simulink model "CrCUI"  (R2016b)
settings: configuration reference "CodeGenConfigSet" (kept outside this file)
values from neighbouring files (symbols this model uses):
  CrCLmp_nLmpTst_C = Calibration.Parameter    [init_CrCUI.m]
  CRCLMP_NORMAL = fi(80,State_uint8)    [init_CrCUI.m]
  CRCLMP_OFF = fi(40,State_uint8)    [init_CrCUI.m]
  CRCLMP_ON = fi(20,State_uint8)    [init_CrCUI.m]
  CrCLmp_tiLmpTstMax_C = Calibration.Parameter    [init_CrCUI.m]
  CrCLmp_tiLmpTstOff_C = Calibration.Parameter    [init_CrCUI.m]
  CrCLmp_tiLmpTstOn_C = Calibration.Parameter    [init_CrCUI.m]
  CRCLMP_VISUAL = fi(10,State_uint8)    [init_CrCUI.m]
  CrCtl_swtAllwSetDrngOvrd_C = Calibration.Parameter    [init_CrCUI.m]
  CrCUI_tiNeutrPosChk_C = Calibration.Parameter    [init_CrCUI.m]
  CrCUI_tiNeutrStr_C = Calibration.Parameter    [init_CrCUI.m]
  CrCUI_tiSwtActvThres_C = Calibration.Parameter    [init_CrCUI.m]
  CrCUI_tiSwtSetThres_C = Calibration.Parameter    [init_CrCUI.m]
undefined symbols (not defined in the file or in its folder): CrCtl_stOpFunc_conv, CrCtl_stShOff_conv, CrCUI_BttnState_conv, CrCUI_DT, CruiseCtl_State_conv, HLSDem_State_conv, Switch_conv, WESDem_State_conv
libraries: CXLib x17, simulink x14
settings Model: Creator=guanxiaoxing  LastModifiedBy=guanxiaoxing
settings ConfigSetRef: SourceLocation=Base Workspace

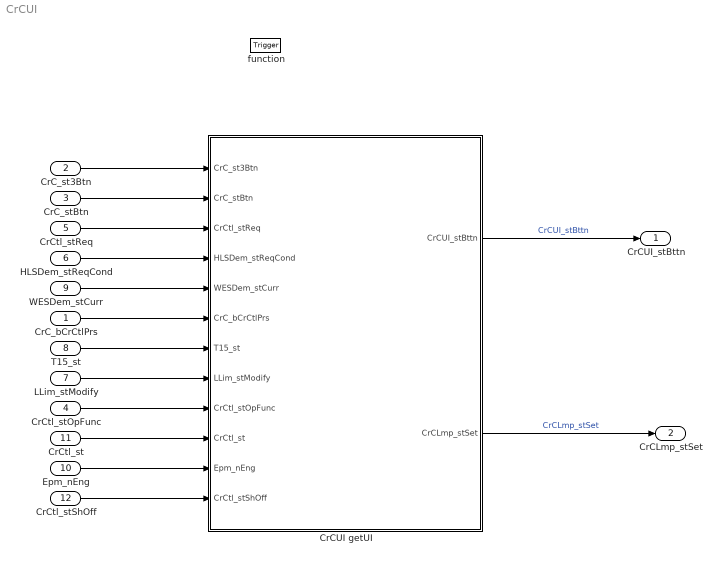
== system CrCUI ==
  CrC_bCrCtlPrs : Inport  Description=Cruise control present status  OutMin=0  OutMax=1  OutDataTypeStr=boolean
  CrC_st3Btn : Inport  Description=two sources for the 3/4 button logic information  Port=2  OutMin=0  OutMax=1  OutDataTypeStr=boolean
  CrC_stBtn : Inport  Description=Status Button Information incase of 3-button logic  Port=3  OutMin=0  OutMax=255  OutDataTypeStr=State_uint8
  CrCtl_stOpFunc : Inport  Description=state of cruise control operation functionality  Port=4  OutDataTypeStr=Enum: CrCtl_stOpFunc_conv
  CrCtl_stReq : Inport  Description=Cruise control is active  Port=5  OutMin=0  OutMax=1  OutDataTypeStr=boolean
  HLSDem_stReqCond : Inport  Description=Status of request for idle speed increase  Port=6  OutMin=0  OutMax=255  OutDataTypeStr=State_uint8
  LLim_stModify : Inport  Description=|  Port=7  OutMin=0  OutMax=1  OutDataTypeStr=boolean
      | Application parameter for Status for changing adjustable
      | vehicle speed limit
  T15_st : Inport  Description=Terminal 15 status after denouncing  Port=8  OutDataTypeStr=Enum: Switch_conv
  WESDem_stCurr : Inport  Description=Status of the working engine Speed Control  Port=9  OutDataTypeStr=Enum: WESDem_State_conv
  Epm_nEng : Inport  Tag=rpm  Description=Engine speed  Port=10  OutMin=0  OutMax=6000  OutDataTypeStr=EngSpeed_rpm
  CrCtl_st : Inport  Description=Application parameter for Cruise Control state  Port=11  OutDataTypeStr=Enum: CruiseCtl_State_conv
  CrCtl_stShOff : Inport  Description=cruise control shut-off requirement  Port=12  OutDataTypeStr=Enum: CrCtl_stShOff_conv
  function : TriggerPort  TriggerType=function-call  VariantControl=Variant
  CrCUI getUI : Subsystem
  CrCUI_stBttn : Outport  Description=Application parameter for status button information  OutDataTypeStr=Enum: CrCUI_BttnState_conv
  CrCLmp_stSet : Outport  Description=input from ASW for cruise set lamp ON/OFF  Port=2  OutMin=0  OutMax=1  OutDataTypeStr=boolean
  wires:
  CrCUI getUI/1(CrCUI_stBttn) -> CrCUI_stBttn/1  "CrCUI_stBttn"
  CrC_st3Btn/1 -> CrCUI getUI/1(CrC_st3Btn)
  CrC_stBtn/1 -> CrCUI getUI/2(CrC_stBtn)
  CrCtl_stReq/1 -> CrCUI getUI/3(CrCtl_stReq)
  HLSDem_stReqCond/1 -> CrCUI getUI/4(HLSDem_stReqCond)
  WESDem_stCurr/1 -> CrCUI getUI/5(WESDem_stCurr)
  T15_st/1 -> CrCUI getUI/7(T15_st)
  CrC_bCrCtlPrs/1 -> CrCUI getUI/6(CrC_bCrCtlPrs)
  CrCtl_stOpFunc/1 -> CrCUI getUI/9(CrCtl_stOpFunc)
  LLim_stModify/1 -> CrCUI getUI/8(LLim_stModify)
  CrCUI getUI/2(CrCLmp_stSet) -> CrCLmp_stSet/1  "CrCLmp_stSet"
  Epm_nEng/1 -> CrCUI getUI/11(Epm_nEng)
  CrCtl_st/1 -> CrCUI getUI/10(CrCtl_st)
  CrCtl_stShOff/1 -> CrCUI getUI/12(CrCtl_stShOff)

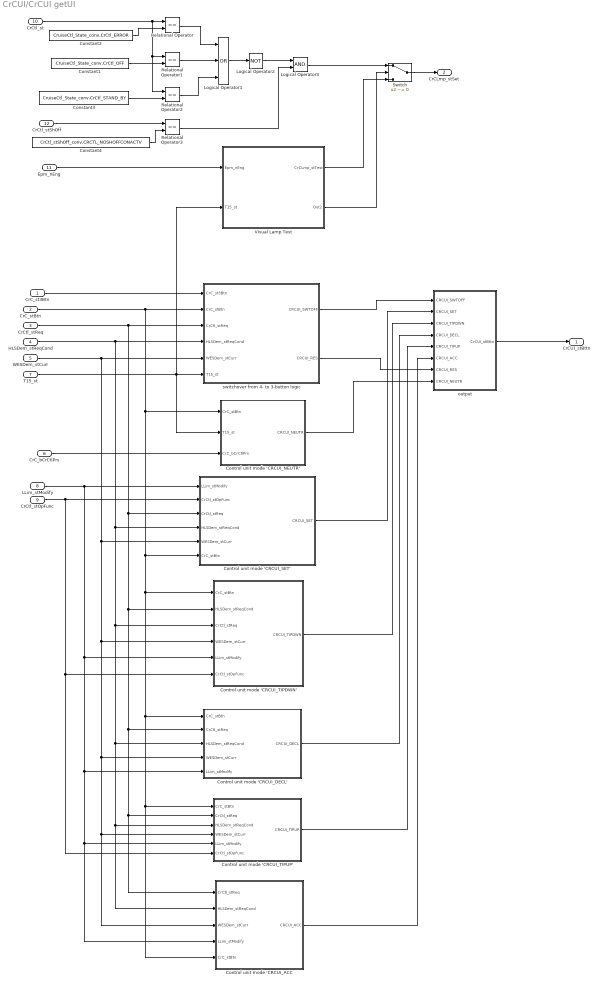
== system CrCUI/CrCUI getUI ==
  CrC_st3Btn : Inport
  CrC_stBtn : Inport  Port=2
  CrCtl_stReq : Inport  Port=3
  HLSDem_stReqCond : Inport  Port=4
  WESDem_stCurr : Inport  Port=5
  CrC_bCrCtlPrs : Inport  Port=6
  T15_st : Inport  Port=7
  LLim_stModify : Inport  Port=8
  CrCtl_stOpFunc : Inport  Port=9
  CrCtl_st : Inport  Port=10
  Epm_nEng : Inport  Port=11
  CrCtl_stShOff : Inport  Port=12
  Constant1 : Constant  Value=CruiseCtl_State_conv.CrCtl_OFF
  Constant2 : Constant  Value=CruiseCtl_State_conv.CrCtl_ERROR
  Constant3 : Constant  Value=CruiseCtl_State_conv.CrCtl_STAND_BY
  Constant4 : Constant  Value=CrCtl_stShOff_conv.CRCTL_NOSHOFFCONACTV
  Control unit mode 'CRCUI_ACC : Subsystem
  Control unit mode 'CRCUI_DECL' : Subsystem
  Control unit mode 'CRCUI_NEUTR' : Subsystem
  Control unit mode 'CRCUI_SET‘ : Subsystem
  Control unit mode 'CRCUI_TIPDWN' : Subsystem
  Control unit mode 'CRCUI_TIPUP' : Subsystem
  Logical Operator1 : Logic  Operator=OR  Inputs=3  AllPortsSameDT=off  OutDataTypeStr=boolean
  Logical Operator2 : Logic  Operator=NOT  AllPortsSameDT=off  OutDataTypeStr=boolean
  Logical Operator3 : Logic  AllPortsSameDT=off  OutDataTypeStr=boolean
  Relational Operator{,1..3} (4 alike) : RelationalOperator  Operator===  OutDataTypeStr=boolean  RndMeth=Simplest
  Switch : Switch  Criteria=u2 ~= 0
  Visual Lamp Test : Subsystem
  output : Subsystem
  switchover from 4- to 3-button logic : Subsystem
  CrCUI_stBttn : Outport
  CrCLmp_stSet : Outport  Port=2
  wires:
  switchover from 4- to 3-button logic/1(CRCUI_SWTOFF) -> output/1(CRCUI_SWTOFF)
  Control unit mode 'CRCUI_SET‘/1(CRCUI_SET) -> output/2(CRCUI_SET)
  Control unit mode 'CRCUI_TIPDWN'/1(CRCUI_TIPDWN) -> output/3(CRCUI_TIPDWN)
  Control unit mode 'CRCUI_DECL'/1(CRCUI_DECL) -> output/4(CRCUI_DECL)
  Control unit mode 'CRCUI_TIPUP'/1(CRCUI_TIPUP) -> output/5(CRCUI_TIPUP)
  Control unit mode 'CRCUI_ACC/1(CRCUI_ACC) -> output/6(CRCUI_ACC)
  switchover from 4- to 3-button logic/2(CRCUI_RES) -> output/7(CRCUI_RES)
  Control unit mode 'CRCUI_NEUTR'/1(CRCUI_NEUTR) -> output/8(CRCUI_NEUTR)
  CrC_st3Btn/1 -> switchover from 4- to 3-button logic/1(CrC_st3Btn)
  CrC_bCrCtlPrs/1 -> Control unit mode 'CRCUI_NEUTR'/3(CrC_bCrCtlPrs)
  CrCtl_stOpFunc/1 -> Control unit mode 'CRCUI_TIPUP'/6(CrCtl_stOpFunc), Control unit mode 'CRCUI_TIPDWN'/6(CrCtl_stOpFunc), Control unit mode 'CRCUI_SET‘/2(CrCtl_stOpFunc)
  LLim_stModify/1 -> Control unit mode 'CRCUI_ACC/4(LLim_stModify), Control unit mode 'CRCUI_TIPUP'/5(LLim_stModify), Control unit mode 'CRCUI_DECL'/5(LLim_stModify), Control unit mode 'CRCUI_TIPDWN'/5(LLim_stModify), Control unit mode 'CRCUI_SET‘/1(LLim_stModify)
  CrCtl_stReq/1 -> Control unit mode 'CRCUI_DECL'/2(CrCtl_stReq), Control unit mode 'CRCUI_TIPUP'/2(CrCtl_stReq), Control unit mode 'CRCUI_ACC/1(CrCtl_stReq), Control unit mode 'CRCUI_TIPDWN'/2(HLSDem_stReqCond), Control unit mode 'CRCUI_SET‘/3(CrCtl_stReq), switchover from 4- to 3-button logic/3(CrCtl_stReq)
  HLSDem_stReqCond/1 -> Control unit mode 'CRCUI_DECL'/3(HLSDem_stReqCond), Control unit mode 'CRCUI_ACC/2(HLSDem_stReqCond), Control unit mode 'CRCUI_TIPUP'/3(HLSDem_stReqCond), Control unit mode 'CRCUI_TIPDWN'/3(CrCtl_stReq), Control unit mode 'CRCUI_SET‘/4(HLSDem_stReqCond), switchover from 4- to 3-button logic/4(HLSDem_stReqCond)
  WESDem_stCurr/1 -> Control unit mode 'CRCUI_ACC/3(WESDem_stCurr), Control unit mode 'CRCUI_TIPUP'/4(WESDem_stCurr), Control unit mode 'CRCUI_DECL'/4(WESDem_stCurr), Control unit mode 'CRCUI_TIPDWN'/4(WESDem_stCurr), Control unit mode 'CRCUI_SET‘/5(WESDem_stCurr), switchover from 4- to 3-button logic/5(WESDem_stCurr)
  CrC_stBtn/1 -> Control unit mode 'CRCUI_DECL'/1(CrC_stBtn), Control unit mode 'CRCUI_ACC/5(CrC_stBtn), Control unit mode 'CRCUI_TIPUP'/1(CrC_stBtn), Control unit mode 'CRCUI_TIPDWN'/1(CrC_stBtn), Control unit mode 'CRCUI_SET‘/6(CrC_stBtn), Control unit mode 'CRCUI_NEUTR'/1(CrC_stBtn), switchover from 4- to 3-button logic/2(CrC_stBtn)
  output/1(CrCUI_stBttn) -> CrCUI_stBttn/1
  Constant1/1 -> Relational Operator1/2
  Constant2/1 -> Relational Operator/2
  Constant3/1 -> Relational Operator2/2
  CrCtl_st/1 -> Relational Operator2/1, Relational Operator1/1, Relational Operator/1
  Relational Operator1/1 -> Logical Operator1/2
  Relational Operator/1 -> Logical Operator1/1
  Relational Operator2/1 -> Logical Operator1/3
  Logical Operator1/1 -> Logical Operator2/1
  Epm_nEng/1 -> Visual Lamp Test/1(Epm_nEng)
  T15_st/1 -> Control unit mode 'CRCUI_NEUTR'/2(T15_st), Visual Lamp Test/2(T15_st), switchover from 4- to 3-button logic/6(T15_st)
  Visual Lamp Test/1(CrCLmp_stTest) -> Switch/3
  Visual Lamp Test/2(Out2) -> Switch/2
  Switch/1 -> CrCLmp_stSet/1
  Logical Operator2/1 -> Logical Operator3/1
  Logical Operator3/1 -> Switch/1
  CrCtl_stShOff/1 -> Relational Operator3/1
  Constant4/1 -> Relational Operator3/2
  Relational Operator3/1 -> Logical Operator3/2

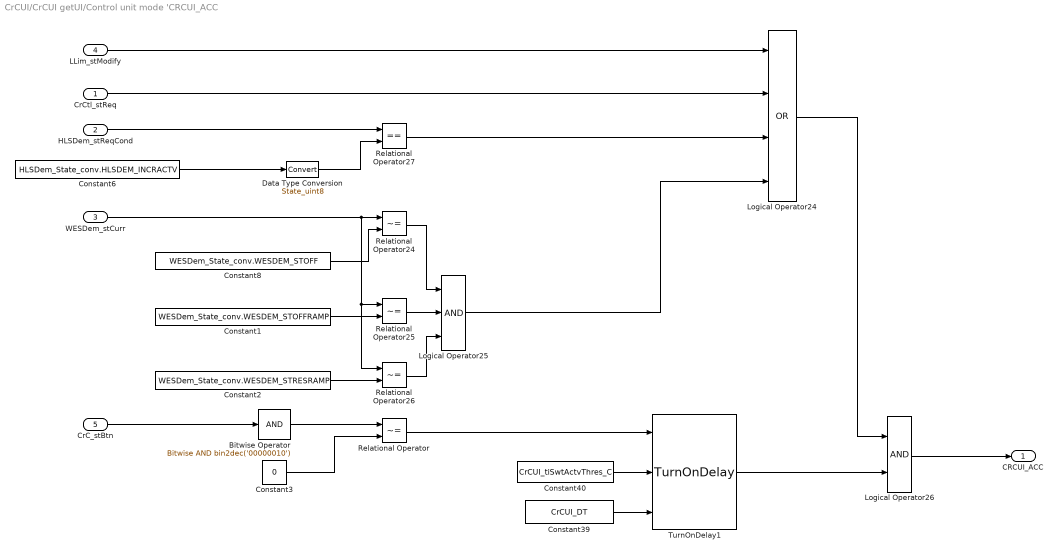
== system CrCUI/CrCUI getUI/Control unit mode 'CRCUI_ACC ==
  CrCtl_stReq : Inport
  HLSDem_stReqCond : Inport  Port=2
  WESDem_stCurr : Inport  Port=3
  LLim_stModify : Inport  Port=4
  CrC_stBtn : Inport  Port=5
  Bitwise Operator : simulink/Logic and Bit Operations/Bitwise Operator  logicop=AND  UseBitMask=on  BitMask=bin2dec('00000010')  BitMaskRealWorld=Stored Integer
  Constant1 : Constant  Value=WESDem_State_conv.WESDEM_STOFFRAMP
  Constant2 : Constant  Value=WESDem_State_conv.WESDEM_STRESRAMP
  Constant3 : Constant  Value=0  OutDataTypeStr=State_uint8
  Constant39 : Constant  Value=CrCUI_DT
  Constant40 : Constant  Value=CrCUI_tiSwtActvThres_C
  Constant6 : Constant  Value=HLSDem_State_conv.HLSDEM_INCRACTV
  Constant8 : Constant  Value=WESDem_State_conv.WESDEM_STOFF
  Data Type Conversion : DataTypeConversion  OutDataTypeStr=State_uint8
  Logical Operator24 : Logic  Operator=OR  Inputs=4  AllPortsSameDT=off  OutDataTypeStr=boolean
  Logical Operator25 : Logic  Inputs=3  AllPortsSameDT=off  OutDataTypeStr=boolean
  Logical Operator26 : Logic  AllPortsSameDT=off  OutDataTypeStr=boolean
  Relational Operator{,24..26} (4 alike) : RelationalOperator  Operator=~=  OutDataTypeStr=boolean  RndMeth=Simplest
  Relational Operator27 : RelationalOperator  Operator===  OutDataTypeStr=boolean  RndMeth=Simplest
  TurnOnDelay1 : CXLib/TurnOnDelay
  CRCUI_ACC : Outport
  wires:
  Constant39/1 -> TurnOnDelay1/3
  Logical Operator26/1 -> CRCUI_ACC/1
  CrCtl_stReq/1 -> Logical Operator24/2
  Relational Operator27/1 -> Logical Operator24/3
  Constant8/1 -> Relational Operator24/2
  Relational Operator25/1 -> Logical Operator25/2
  Logical Operator25/1 -> Logical Operator24/4
  WESDem_stCurr/1 -> Relational Operator26/1, Relational Operator25/1, Relational Operator24/1
  HLSDem_stReqCond/1 -> Relational Operator27/1
  Constant1/1 -> Relational Operator25/2
  Relational Operator26/1 -> Logical Operator25/3
  Relational Operator/1 -> TurnOnDelay1/1
  Constant2/1 -> Relational Operator26/2
  TurnOnDelay1/1 -> Logical Operator26/2
  Constant40/1 -> TurnOnDelay1/2
  Relational Operator24/1 -> Logical Operator25/1
  Constant6/1 -> Data Type Conversion/1
  Logical Operator24/1 -> Logical Operator26/1
  CrC_stBtn/1 -> Bitwise Operator/1
  LLim_stModify/1 -> Logical Operator24/1
  Bitwise Operator/1 -> Relational Operator/1
  Constant3/1 -> Relational Operator/2
  Data Type Conversion/1 -> Relational Operator27/2

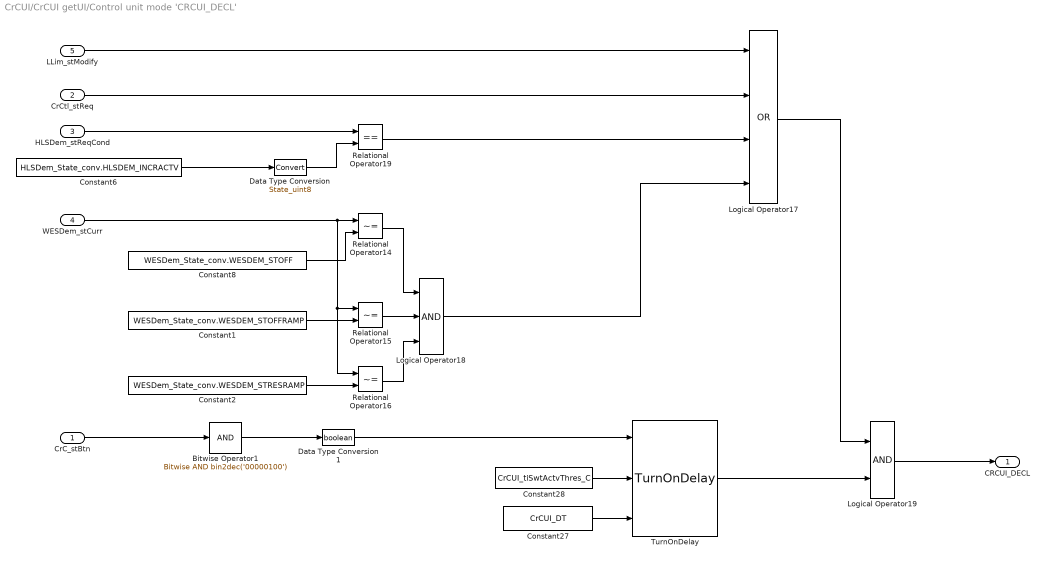
== system CrCUI/CrCUI getUI/Control unit mode 'CRCUI_DECL' ==
  CrC_stBtn : Inport
  CrCtl_stReq : Inport  Port=2
  HLSDem_stReqCond : Inport  Port=3
  WESDem_stCurr : Inport  Port=4
  LLim_stModify : Inport  Port=5
  Bitwise Operator1 : simulink/Logic and Bit Operations/Bitwise Operator  logicop=AND  UseBitMask=on  BitMask=bin2dec('00000100')  BitMaskRealWorld=Stored Integer
  Constant1 : Constant  Value=WESDem_State_conv.WESDEM_STOFFRAMP
  Constant2 : Constant  Value=WESDem_State_conv.WESDEM_STRESRAMP
  Constant27 : Constant  Value=CrCUI_DT
  Constant28 : Constant  Value=CrCUI_tiSwtActvThres_C
  Constant6 : Constant  Value=HLSDem_State_conv.HLSDEM_INCRACTV
  Constant8 : Constant  Value=WESDem_State_conv.WESDEM_STOFF
  Data Type Conversion : DataTypeConversion  OutDataTypeStr=State_uint8
  Data Type Conversion1 : DataTypeConversion  OutDataTypeStr=boolean
  Logical Operator17 : Logic  Operator=OR  Inputs=4  AllPortsSameDT=off  OutDataTypeStr=boolean
  Logical Operator18 : Logic  Inputs=3  AllPortsSameDT=off  OutDataTypeStr=boolean
  Logical Operator19 : Logic  AllPortsSameDT=off  OutDataTypeStr=boolean
  Relational Operator14 : RelationalOperator  Operator=~=  OutDataTypeStr=boolean  RndMeth=Simplest
  Relational Operator15 : RelationalOperator  Operator=~=  OutDataTypeStr=boolean  RndMeth=Simplest
  Relational Operator16 : RelationalOperator  Operator=~=  OutDataTypeStr=boolean  RndMeth=Simplest
  Relational Operator19 : RelationalOperator  Operator===  OutDataTypeStr=boolean  RndMeth=Simplest
  TurnOnDelay : CXLib/TurnOnDelay
  CRCUI_DECL : Outport
  wires:
  CrCtl_stReq/1 -> Logical Operator17/2
  Relational Operator19/1 -> Logical Operator17/3
  HLSDem_stReqCond/1 -> Relational Operator19/1
  Constant6/1 -> Data Type Conversion/1
  Constant1/1 -> Relational Operator15/2
  Logical Operator18/1 -> Logical Operator17/4
  Constant2/1 -> Relational Operator16/2
  Relational Operator16/1 -> Logical Operator18/3
  Logical Operator19/1 -> CRCUI_DECL/1
  Constant27/1 -> TurnOnDelay/3
  Constant8/1 -> Relational Operator14/2
  Relational Operator14/1 -> Logical Operator18/1
  Bitwise Operator1/1 -> Data Type Conversion1/1
  Logical Operator17/1 -> Logical Operator19/1
  WESDem_stCurr/1 -> Relational Operator16/1, Relational Operator15/1, Relational Operator14/1
  Relational Operator15/1 -> Logical Operator18/2
  TurnOnDelay/1 -> Logical Operator19/2
  Constant28/1 -> TurnOnDelay/2
  CrC_stBtn/1 -> Bitwise Operator1/1
  LLim_stModify/1 -> Logical Operator17/1
  Data Type Conversion/1 -> Relational Operator19/2
  Data Type Conversion1/1 -> TurnOnDelay/1

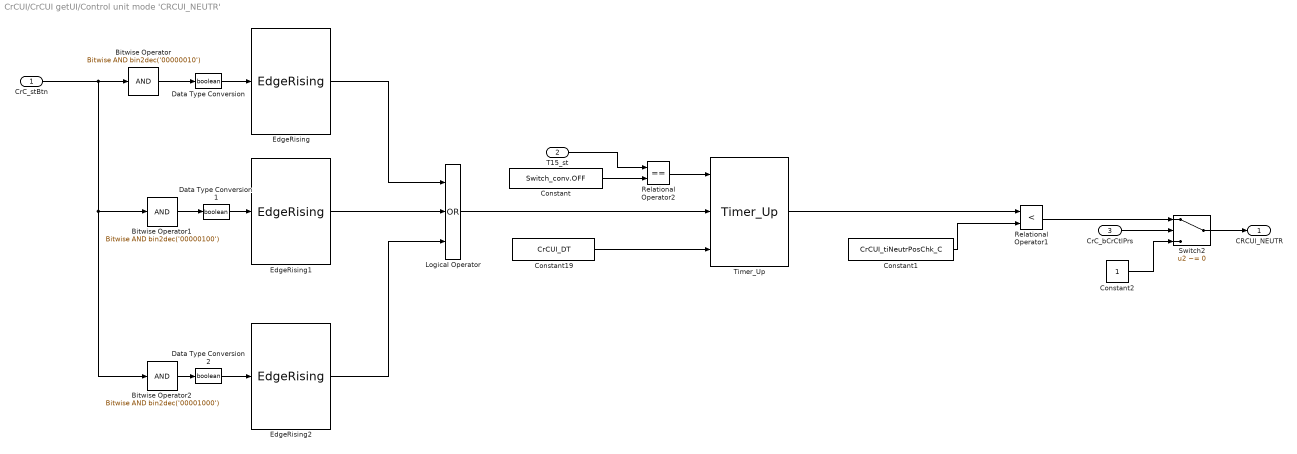
== system CrCUI/CrCUI getUI/Control unit mode 'CRCUI_NEUTR' ==
  CrC_stBtn : Inport
  T15_st : Inport  Port=2
  CrC_bCrCtlPrs : Inport  Port=3
  Bitwise Operator : simulink/Logic and Bit Operations/Bitwise Operator  logicop=AND  UseBitMask=on  BitMask=bin2dec('00000010')  BitMaskRealWorld=Stored Integer
  Bitwise Operator1 : simulink/Logic and Bit Operations/Bitwise Operator  logicop=AND  UseBitMask=on  BitMask=bin2dec('00000100')  BitMaskRealWorld=Stored Integer
  Bitwise Operator2 : simulink/Logic and Bit Operations/Bitwise Operator  logicop=AND  UseBitMask=on  BitMask=bin2dec('00001000')  BitMaskRealWorld=Stored Integer
  Constant : Constant  Value=Switch_conv.OFF
  Constant1 : Constant  Value=CrCUI_tiNeutrPosChk_C
  Constant19 : Constant  Value=CrCUI_DT
  Constant2 : Constant  OutDataTypeStr=boolean
  Data Type Conversion : DataTypeConversion  OutDataTypeStr=boolean
  Data Type Conversion1 : DataTypeConversion  OutDataTypeStr=boolean
  Data Type Conversion2 : DataTypeConversion  OutDataTypeStr=boolean
  EdgeRising : CXLib/EdgeRising
  EdgeRising1 : CXLib/EdgeRising
  EdgeRising2 : CXLib/EdgeRising
  Logical Operator : Logic  Operator=OR  Inputs=3  AllPortsSameDT=off  OutDataTypeStr=boolean
  Relational Operator1 : RelationalOperator  Operator=<  OutDataTypeStr=boolean  RndMeth=Simplest
  Relational Operator2 : RelationalOperator  Operator===  OutDataTypeStr=boolean  RndMeth=Simplest
  Switch2 : Switch  Criteria=u2 ~= 0
  Timer_Up : CXLib/Timer_Up
  CRCUI_NEUTR : Outport
  wires:
  CrC_stBtn/1 -> Bitwise Operator1/1, Bitwise Operator2/1, Bitwise Operator/1
  Bitwise Operator/1 -> Data Type Conversion/1
  Bitwise Operator1/1 -> Data Type Conversion1/1
  Bitwise Operator2/1 -> Data Type Conversion2/1
  EdgeRising1/1 -> Logical Operator/2
  EdgeRising/1 -> Logical Operator/1
  EdgeRising2/1 -> Logical Operator/3
  Logical Operator/1 -> Timer_Up/2
  Constant19/1 -> Timer_Up/3
  Constant1/1 -> Relational Operator1/2
  Data Type Conversion/1 -> EdgeRising/1
  Data Type Conversion1/1 -> EdgeRising1/1
  Data Type Conversion2/1 -> EdgeRising2/1
  Relational Operator2/1 -> Timer_Up/1
  Constant/1 -> Relational Operator2/2
  T15_st/1 -> Relational Operator2/1
  Timer_Up/1 -> Relational Operator1/1
  CrC_bCrCtlPrs/1 -> Switch2/2
  Relational Operator1/1 -> Switch2/1
  Switch2/1 -> CRCUI_NEUTR/1
  Constant2/1 -> Switch2/3

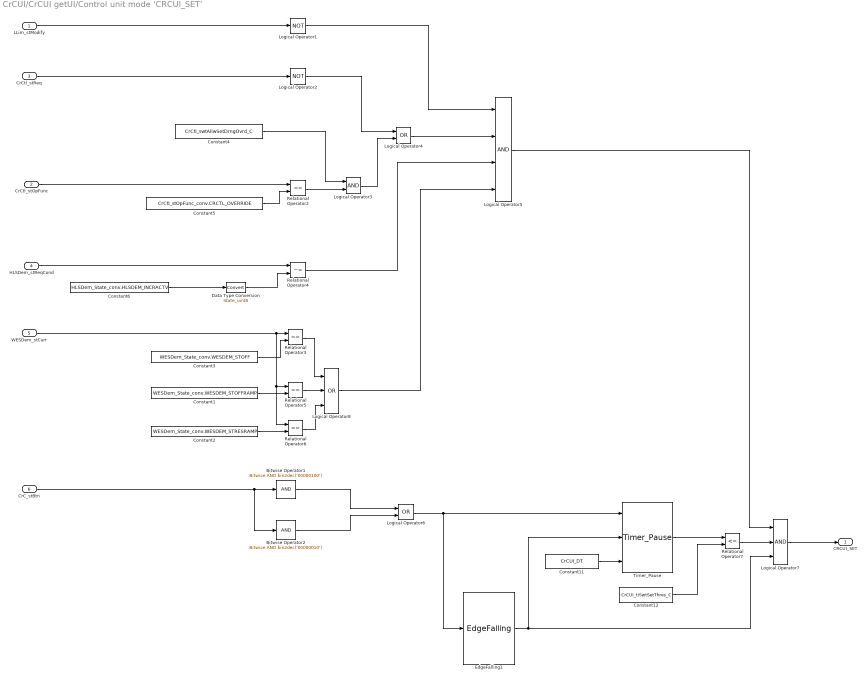
== system CrCUI/CrCUI getUI/Control unit mode 'CRCUI_SET‘ ==
  LLim_stModify : Inport
  CrCtl_stOpFunc : Inport  Port=2
  CrCtl_stReq : Inport  Port=3
  HLSDem_stReqCond : Inport  Port=4
  WESDem_stCurr : Inport  Port=5
  CrC_stBtn : Inport  Port=6
  Bitwise Operator1 : simulink/Logic and Bit Operations/Bitwise Operator  logicop=AND  UseBitMask=on  BitMask=bin2dec('00000100')  BitMaskRealWorld=Stored Integer
  Bitwise Operator2 : simulink/Logic and Bit Operations/Bitwise Operator  logicop=AND  UseBitMask=on  BitMask=bin2dec('00000010')  BitMaskRealWorld=Stored Integer
  Constant1 : Constant  Value=WESDem_State_conv.WESDEM_STOFFRAMP
  Constant11 : Constant  Value=CrCUI_DT
  Constant12 : Constant  Value=CrCUI_tiSwtSetThres_C
  Constant2 : Constant  Value=WESDem_State_conv.WESDEM_STRESRAMP
  Constant3 : Constant  Value=WESDem_State_conv.WESDEM_STOFF
  Constant4 : Constant  Value=CrCtl_swtAllwSetDrngOvrd_C
  Constant5 : Constant  Value=CrCtl_stOpFunc_conv.CRCTL_OVERRIDE
  Constant6 : Constant  Value=HLSDem_State_conv.HLSDEM_INCRACTV
  Data Type Conversion : DataTypeConversion  OutDataTypeStr=State_uint8
  EdgeFalling1 : CXLib/EdgeFalling
  Logical Operator1 : Logic  Operator=NOT  AllPortsSameDT=off  OutDataTypeStr=boolean
  Logical Operator2 : Logic  Operator=NOT  AllPortsSameDT=off  OutDataTypeStr=boolean
  Logical Operator3 : Logic  AllPortsSameDT=off  OutDataTypeStr=boolean
  Logical Operator4 : Logic  Operator=OR  AllPortsSameDT=off  OutDataTypeStr=boolean
  Logical Operator5 : Logic  Inputs=4  AllPortsSameDT=off  OutDataTypeStr=boolean
  Logical Operator6 : Logic  Operator=OR  AllPortsSameDT=off  OutDataTypeStr=boolean
  Logical Operator7 : Logic  Inputs=3  AllPortsSameDT=off  OutDataTypeStr=boolean
  Logical Operator8 : Logic  Operator=OR  Inputs=3  AllPortsSameDT=off  OutDataTypeStr=boolean
  Relational Operator{2..3,5..6} (4 alike) : RelationalOperator  Operator===  OutDataTypeStr=boolean  RndMeth=Simplest
  Relational Operator4 : RelationalOperator  Operator=~=  OutDataTypeStr=boolean  RndMeth=Simplest
  Relational Operator7 : RelationalOperator  Operator=<=  OutDataTypeStr=boolean  RndMeth=Simplest
  Timer_Pause : CXLib/Timer_Pause
  CRCUI_SET : Outport
  wires:
  CrCtl_stOpFunc/1 -> Relational Operator2/1
  Logical Operator2/1 -> Logical Operator4/1
  Logical Operator3/1 -> Logical Operator4/2
  Constant6/1 -> Data Type Conversion/1
  Relational Operator2/1 -> Logical Operator3/2
  LLim_stModify/1 -> Logical Operator1/1
  CrCtl_stReq/1 -> Logical Operator2/1
  Constant5/1 -> Relational Operator2/2
  Constant4/1 -> Logical Operator3/1
  HLSDem_stReqCond/1 -> Relational Operator4/1
  Relational Operator4/1 -> Logical Operator5/3
  Bitwise Operator2/1 -> Logical Operator6/2
  Constant3/1 -> Relational Operator3/2
  EdgeFalling1/1 -> Timer_Pause/2, Logical Operator7/3
  Constant11/1 -> Timer_Pause/3
  Logical Operator6/1 -> Timer_Pause/1, EdgeFalling1/1
  Logical Operator4/1 -> Logical Operator5/2
  Logical Operator7/1 -> CRCUI_SET/1
  WESDem_stCurr/1 -> Relational Operator6/1, Relational Operator5/1, Relational Operator3/1
  Constant1/1 -> Relational Operator5/2
  Relational Operator3/1 -> Logical Operator8/1
  CrC_stBtn/1 -> Bitwise Operator2/1, Bitwise Operator1/1
  Logical Operator5/1 -> Logical Operator7/1
  Relational Operator5/1 -> Logical Operator8/2
  Relational Operator6/1 -> Logical Operator8/3
  Logical Operator8/1 -> Logical Operator5/4
  Constant12/1 -> Relational Operator7/2
  Timer_Pause/1 -> Relational Operator7/1
  Relational Operator7/1 -> Logical Operator7/2
  Bitwise Operator1/1 -> Logical Operator6/1
  Logical Operator1/1 -> Logical Operator5/1
  Constant2/1 -> Relational Operator6/2
  Data Type Conversion/1 -> Relational Operator4/2

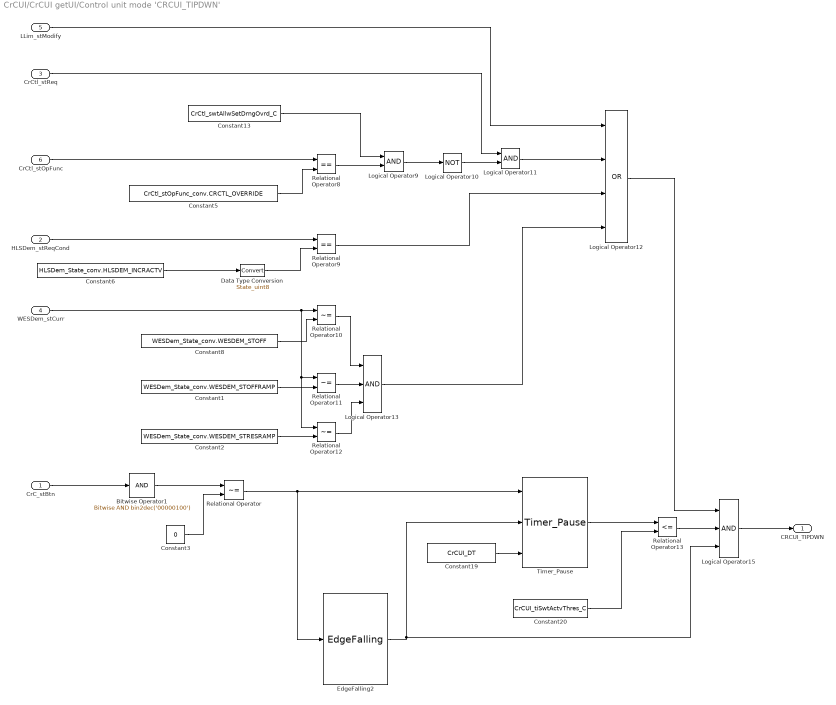
== system CrCUI/CrCUI getUI/Control unit mode 'CRCUI_TIPDWN' ==
  CrC_stBtn : Inport
  HLSDem_stReqCond : Inport  Port=2
  CrCtl_stReq : Inport  Port=3
  WESDem_stCurr : Inport  Port=4
  LLim_stModify : Inport  Port=5
  CrCtl_stOpFunc : Inport  Port=6
  Bitwise Operator1 : simulink/Logic and Bit Operations/Bitwise Operator  logicop=AND  UseBitMask=on  BitMask=bin2dec('00000100')  BitMaskRealWorld=Stored Integer
  Constant1 : Constant  Value=WESDem_State_conv.WESDEM_STOFFRAMP
  Constant13 : Constant  Value=CrCtl_swtAllwSetDrngOvrd_C
  Constant19 : Constant  Value=CrCUI_DT
  Constant2 : Constant  Value=WESDem_State_conv.WESDEM_STRESRAMP
  Constant20 : Constant  Value=CrCUI_tiSwtActvThres_C
  Constant3 : Constant  Value=0  OutDataTypeStr=uint16
  Constant5 : Constant  Value=CrCtl_stOpFunc_conv.CRCTL_OVERRIDE
  Constant6 : Constant  Value=HLSDem_State_conv.HLSDEM_INCRACTV
  Constant8 : Constant  Value=WESDem_State_conv.WESDEM_STOFF
  Data Type Conversion : DataTypeConversion  OutDataTypeStr=State_uint8
  EdgeFalling2 : CXLib/EdgeFalling
  Logical Operator10 : Logic  Operator=NOT  AllPortsSameDT=off  OutDataTypeStr=boolean
  Logical Operator11 : Logic  AllPortsSameDT=off  OutDataTypeStr=boolean
  Logical Operator12 : Logic  Operator=OR  Inputs=4  AllPortsSameDT=off  OutDataTypeStr=boolean
  Logical Operator13 : Logic  Inputs=3  AllPortsSameDT=off  OutDataTypeStr=boolean
  Logical Operator15 : Logic  Inputs=3  AllPortsSameDT=off  OutDataTypeStr=boolean
  Logical Operator9 : Logic  AllPortsSameDT=off  OutDataTypeStr=boolean
  Relational Operator{,10..12} (4 alike) : RelationalOperator  Operator=~=  OutDataTypeStr=boolean  RndMeth=Simplest
  Relational Operator13 : RelationalOperator  Operator=<=  OutDataTypeStr=boolean  RndMeth=Simplest
  Relational Operator8 : RelationalOperator  Operator===  OutDataTypeStr=boolean  RndMeth=Simplest
  Relational Operator9 : RelationalOperator  Operator===  OutDataTypeStr=boolean  RndMeth=Simplest
  Timer_Pause : CXLib/Timer_Pause
  CRCUI_TIPDWN : Outport
  wires:
  Constant5/1 -> Relational Operator8/2
  CrCtl_stOpFunc/1 -> Relational Operator8/1
  Constant13/1 -> Logical Operator9/1
  Logical Operator9/1 -> Logical Operator10/1
  Logical Operator10/1 -> Logical Operator11/2
  Relational Operator8/1 -> Logical Operator9/2
  CrCtl_stReq/1 -> Logical Operator11/1
  Relational Operator/1 -> EdgeFalling2/1, Timer_Pause/1
  HLSDem_stReqCond/1 -> Relational Operator9/1
  WESDem_stCurr/1 -> Relational Operator12/1, Relational Operator11/1, Relational Operator10/1
  Relational Operator10/1 -> Logical Operator13/1
  Constant19/1 -> Timer_Pause/3
  Relational Operator11/1 -> Logical Operator13/2
  Constant20/1 -> Relational Operator13/2
  Relational Operator9/1 -> Logical Operator12/3
  Timer_Pause/1 -> Relational Operator13/1
  Relational Operator13/1 -> Logical Operator15/2
  Logical Operator12/1 -> Logical Operator15/1
  Logical Operator15/1 -> CRCUI_TIPDWN/1
  Constant6/1 -> Data Type Conversion/1
  Constant2/1 -> Relational Operator12/2
  EdgeFalling2/1 -> Timer_Pause/2, Logical Operator15/3
  Constant8/1 -> Relational Operator10/2
  Logical Operator13/1 -> Logical Operator12/4
  Logical Operator11/1 -> Logical Operator12/2
  Relational Operator12/1 -> Logical Operator13/3
  Constant1/1 -> Relational Operator11/2
  CrC_stBtn/1 -> Bitwise Operator1/1
  LLim_stModify/1 -> Logical Operator12/1
  Constant3/1 -> Relational Operator/2
  Bitwise Operator1/1 -> Relational Operator/1
  Data Type Conversion/1 -> Relational Operator9/2

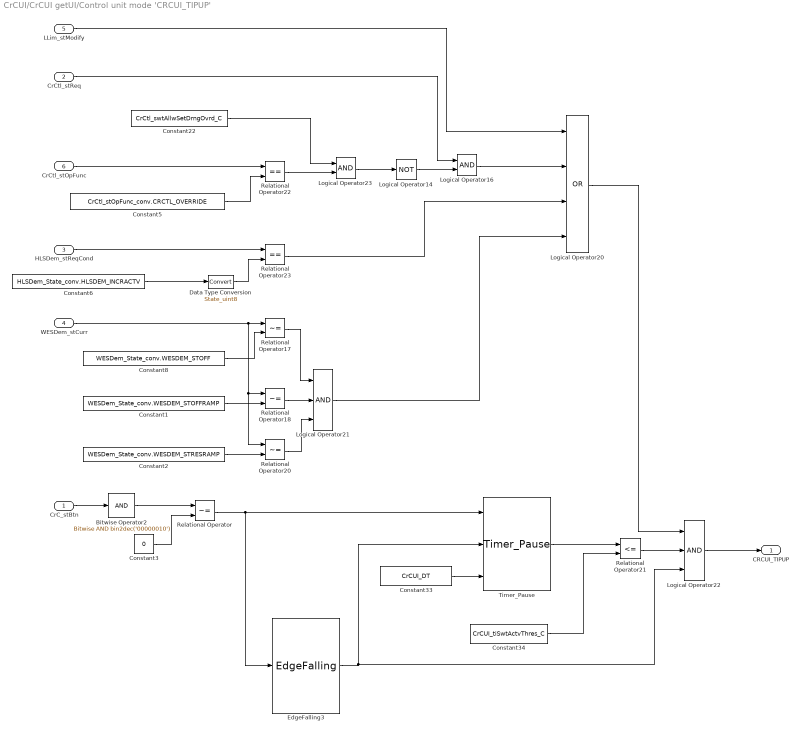
== system CrCUI/CrCUI getUI/Control unit mode 'CRCUI_TIPUP' ==
  CrC_stBtn : Inport
  CrCtl_stReq : Inport  Port=2
  HLSDem_stReqCond : Inport  Port=3
  WESDem_stCurr : Inport  Port=4
  LLim_stModify : Inport  Port=5
  CrCtl_stOpFunc : Inport  Port=6
  Bitwise Operator2 : simulink/Logic and Bit Operations/Bitwise Operator  logicop=AND  UseBitMask=on  BitMask=bin2dec('00000010')  BitMaskRealWorld=Stored Integer
  Constant1 : Constant  Value=WESDem_State_conv.WESDEM_STOFFRAMP
  Constant2 : Constant  Value=WESDem_State_conv.WESDEM_STRESRAMP
  Constant22 : Constant  Value=CrCtl_swtAllwSetDrngOvrd_C
  Constant3 : Constant  Value=0  OutDataTypeStr=State_uint8
  Constant33 : Constant  Value=CrCUI_DT
  Constant34 : Constant  Value=CrCUI_tiSwtActvThres_C
  Constant5 : Constant  Value=CrCtl_stOpFunc_conv.CRCTL_OVERRIDE
  Constant6 : Constant  Value=HLSDem_State_conv.HLSDEM_INCRACTV
  Constant8 : Constant  Value=WESDem_State_conv.WESDEM_STOFF
  Data Type Conversion : DataTypeConversion  OutDataTypeStr=State_uint8
  EdgeFalling3 : CXLib/EdgeFalling
  Logical Operator14 : Logic  Operator=NOT  AllPortsSameDT=off  OutDataTypeStr=boolean
  Logical Operator16 : Logic  AllPortsSameDT=off  OutDataTypeStr=boolean
  Logical Operator20 : Logic  Operator=OR  Inputs=4  AllPortsSameDT=off  OutDataTypeStr=boolean
  Logical Operator21 : Logic  Inputs=3  AllPortsSameDT=off  OutDataTypeStr=boolean
  Logical Operator22 : Logic  Inputs=3  AllPortsSameDT=off  OutDataTypeStr=boolean
  Logical Operator23 : Logic  AllPortsSameDT=off  OutDataTypeStr=boolean
  Relational Operator{,17..18,20} (4 alike) : RelationalOperator  Operator=~=  OutDataTypeStr=boolean  RndMeth=Simplest
  Relational Operator21 : RelationalOperator  Operator=<=  OutDataTypeStr=boolean  RndMeth=Simplest
  Relational Operator22 : RelationalOperator  Operator===  OutDataTypeStr=boolean  RndMeth=Simplest
  Relational Operator23 : RelationalOperator  Operator===  OutDataTypeStr=boolean  RndMeth=Simplest
  Timer_Pause : CXLib/Timer_Pause
  CRCUI_TIPUP : Outport
  wires:
  Logical Operator16/1 -> Logical Operator20/2
  Constant5/1 -> Relational Operator22/2
  WESDem_stCurr/1 -> Relational Operator20/1, Relational Operator18/1, Relational Operator17/1
  Relational Operator17/1 -> Logical Operator21/1
  Logical Operator14/1 -> Logical Operator16/2
  CrCtl_stReq/1 -> Logical Operator16/1
  Constant6/1 -> Data Type Conversion/1
  Logical Operator23/1 -> Logical Operator14/1
  Relational Operator22/1 -> Logical Operator23/2
  Constant1/1 -> Relational Operator18/2
  Relational Operator18/1 -> Logical Operator21/2
  Relational Operator23/1 -> Logical Operator20/3
  CrCtl_stOpFunc/1 -> Relational Operator22/1
  HLSDem_stReqCond/1 -> Relational Operator23/1
  Relational Operator20/1 -> Logical Operator21/3
  Constant22/1 -> Logical Operator23/1
  Constant8/1 -> Relational Operator17/2
  Constant34/1 -> Relational Operator21/2
  Constant2/1 -> Relational Operator20/2
  Logical Operator20/1 -> Logical Operator22/1
  Logical Operator22/1 -> CRCUI_TIPUP/1
  Constant33/1 -> Timer_Pause/3
  Relational Operator21/1 -> Logical Operator22/2
  Timer_Pause/1 -> Relational Operator21/1
  Logical Operator21/1 -> Logical Operator20/4
  EdgeFalling3/1 -> Timer_Pause/2, Logical Operator22/3
  Relational Operator/1 -> EdgeFalling3/1, Timer_Pause/1
  CrC_stBtn/1 -> Bitwise Operator2/1
  LLim_stModify/1 -> Logical Operator20/1
  Constant3/1 -> Relational Operator/2
  Bitwise Operator2/1 -> Relational Operator/1
  Data Type Conversion/1 -> Relational Operator23/2

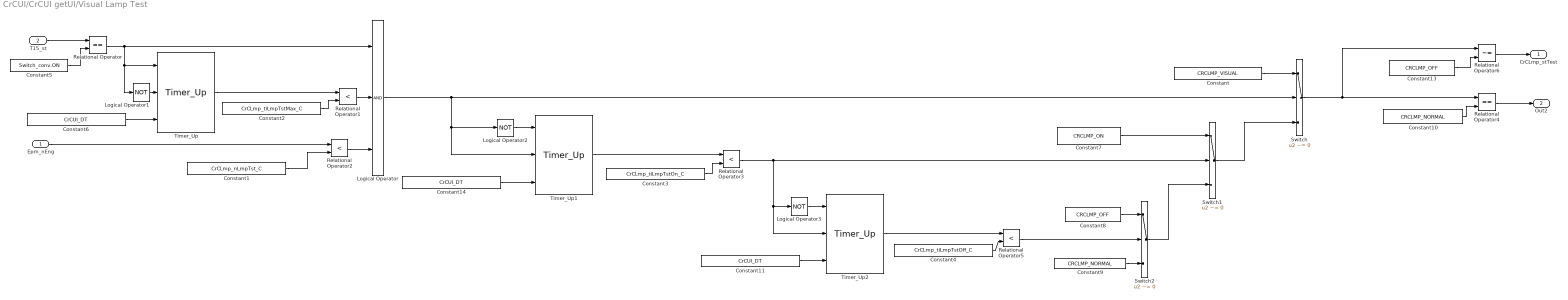
== system CrCUI/CrCUI getUI/Visual Lamp Test ==
  Epm_nEng : Inport
  T15_st : Inport  Port=2
  Constant : Constant  Value=CRCLMP_VISUAL
  Constant1 : Constant  Value=CrCLmp_nLmpTst_C
  Constant10 : Constant  Value=CRCLMP_NORMAL
  Constant11 : Constant  Value=CrCUI_DT
  Constant13 : Constant  Value=CRCLMP_OFF
  Constant14 : Constant  Value=CrCUI_DT
  Constant2 : Constant  Value=CrCLmp_tiLmpTstMax_C
  Constant3 : Constant  Value=CrCLmp_tiLmpTstOn_C
  Constant4 : Constant  Value=CrCLmp_tiLmpTstOff_C
  Constant5 : Constant  Value=Switch_conv.ON
  Constant6 : Constant  Value=CrCUI_DT
  Constant7 : Constant  Value=CRCLMP_ON
  Constant8 : Constant  Value=CRCLMP_OFF
  Constant9 : Constant  Value=CRCLMP_NORMAL
  Logical Operator : Logic  Inputs=3  AllPortsSameDT=off  OutDataTypeStr=boolean
  Logical Operator1 : Logic  Operator=NOT  AllPortsSameDT=off  OutDataTypeStr=boolean
  Logical Operator2 : Logic  Operator=NOT  AllPortsSameDT=off  OutDataTypeStr=boolean
  Logical Operator3 : Logic  Operator=NOT  AllPortsSameDT=off  OutDataTypeStr=boolean
  Relational Operator : RelationalOperator  Operator===  OutDataTypeStr=boolean  RndMeth=Simplest
  Relational Operator{1..3,5} (4 alike) : RelationalOperator  Operator=<  OutDataTypeStr=boolean  RndMeth=Simplest
  Relational Operator4 : RelationalOperator  Operator===  OutDataTypeStr=boolean  RndMeth=Simplest
  Relational Operator6 : RelationalOperator  Operator=~=  OutDataTypeStr=boolean  RndMeth=Simplest
  Switch : Switch  Criteria=u2 ~= 0
  Switch1 : Switch  Criteria=u2 ~= 0
  Switch2 : Switch  Criteria=u2 ~= 0
  Timer_Up : CXLib/Timer_Up
  Timer_Up1 : CXLib/Timer_Up
  Timer_Up2 : CXLib/Timer_Up
  CrCLmp_stTest : Outport
  Out2 : Outport  Port=2
  wires:
  T15_st/1 -> Relational Operator/1
  Constant5/1 -> Relational Operator/2
  Relational Operator/1 -> Logical Operator/1, Logical Operator1/1, Timer_Up/1
  Constant6/1 -> Timer_Up/3
  Logical Operator1/1 -> Timer_Up/2
  Timer_Up/1 -> Relational Operator1/1
  Relational Operator1/1 -> Logical Operator/2
  Constant2/1 -> Relational Operator1/2
  Relational Operator2/1 -> Logical Operator/3
  Epm_nEng/1 -> Relational Operator2/1
  Constant1/1 -> Relational Operator2/2
  Logical Operator/1 -> Timer_Up1/2, Logical Operator2/1, Switch/2
  Constant/1 -> Switch/1
  Switch1/1 -> Switch/3
  Constant7/1 -> Switch1/1
  Switch2/1 -> Switch1/3
  Constant8/1 -> Switch2/1
  Constant9/1 -> Switch2/3
  Relational Operator4/1 -> Out2/1
  Constant10/1 -> Relational Operator4/2
  Logical Operator2/1 -> Timer_Up1/1
  Timer_Up1/1 -> Relational Operator3/1
  Constant14/1 -> Timer_Up1/3
  Constant3/1 -> Relational Operator3/2
  Relational Operator5/1 -> Switch2/2
  Constant4/1 -> Relational Operator5/2
  Timer_Up2/1 -> Relational Operator5/1
  Constant11/1 -> Timer_Up2/3
  Relational Operator3/1 -> Timer_Up2/2, Logical Operator3/1, Switch1/2
  Logical Operator3/1 -> Timer_Up2/1
  Switch/1 -> Relational Operator6/1, Relational Operator4/1
  Constant13/1 -> Relational Operator6/2
  Relational Operator6/1 -> CrCLmp_stTest/1

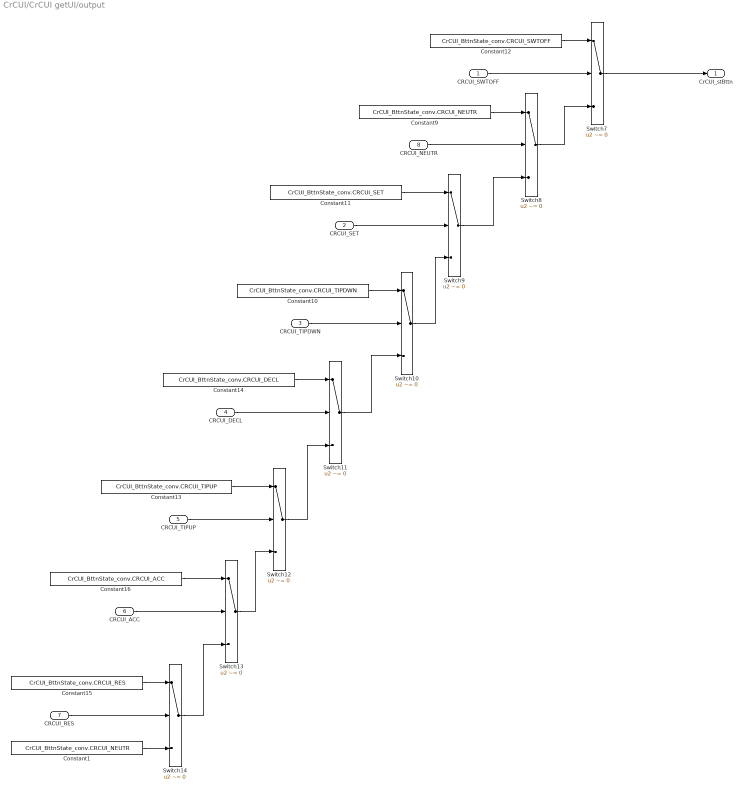
== system CrCUI/CrCUI getUI/output ==
  CRCUI_SWTOFF : Inport
  CRCUI_SET : Inport  Port=2
  CRCUI_TIPDWN : Inport  Port=3
  CRCUI_DECL : Inport  Port=4
  CRCUI_TIPUP : Inport  Port=5
  CRCUI_ACC : Inport  Port=6
  CRCUI_RES : Inport  Port=7
  CRCUI_NEUTR : Inport  Port=8
  Constant1 : Constant  Value=CrCUI_BttnState_conv.CRCUI_NEUTR
  Constant10 : Constant  Value=CrCUI_BttnState_conv.CRCUI_TIPDWN
  Constant11 : Constant  Value=CrCUI_BttnState_conv.CRCUI_SET
  Constant12 : Constant  Value=CrCUI_BttnState_conv.CRCUI_SWTOFF
  Constant13 : Constant  Value=CrCUI_BttnState_conv.CRCUI_TIPUP
  Constant14 : Constant  Value=CrCUI_BttnState_conv.CRCUI_DECL
  Constant15 : Constant  Value=CrCUI_BttnState_conv.CRCUI_RES
  Constant16 : Constant  Value=CrCUI_BttnState_conv.CRCUI_ACC
  Constant9 : Constant  Value=CrCUI_BttnState_conv.CRCUI_NEUTR
  Switch{7..14} (8 alike) : Switch  Criteria=u2 ~= 0
  CrCUI_stBttn : Outport
  wires:
  CRCUI_SWTOFF/1 -> Switch7/2
  Constant12/1 -> Switch7/1
  Switch8/1 -> Switch7/3
  CRCUI_NEUTR/1 -> Switch8/2
  Constant9/1 -> Switch8/1
  Switch9/1 -> Switch8/3
  CRCUI_SET/1 -> Switch9/2
  Constant11/1 -> Switch9/1
  Switch10/1 -> Switch9/3
  CRCUI_TIPDWN/1 -> Switch10/2
  Constant10/1 -> Switch10/1
  Switch11/1 -> Switch10/3
  CRCUI_DECL/1 -> Switch11/2
  Constant14/1 -> Switch11/1
  Switch12/1 -> Switch11/3
  CRCUI_TIPUP/1 -> Switch12/2
  Constant13/1 -> Switch12/1
  Switch13/1 -> Switch12/3
  CRCUI_ACC/1 -> Switch13/2
  Constant16/1 -> Switch13/1
  Switch14/1 -> Switch13/3
  CRCUI_RES/1 -> Switch14/2
  Constant15/1 -> Switch14/1
  Switch7/1 -> CrCUI_stBttn/1
  Constant1/1 -> Switch14/3

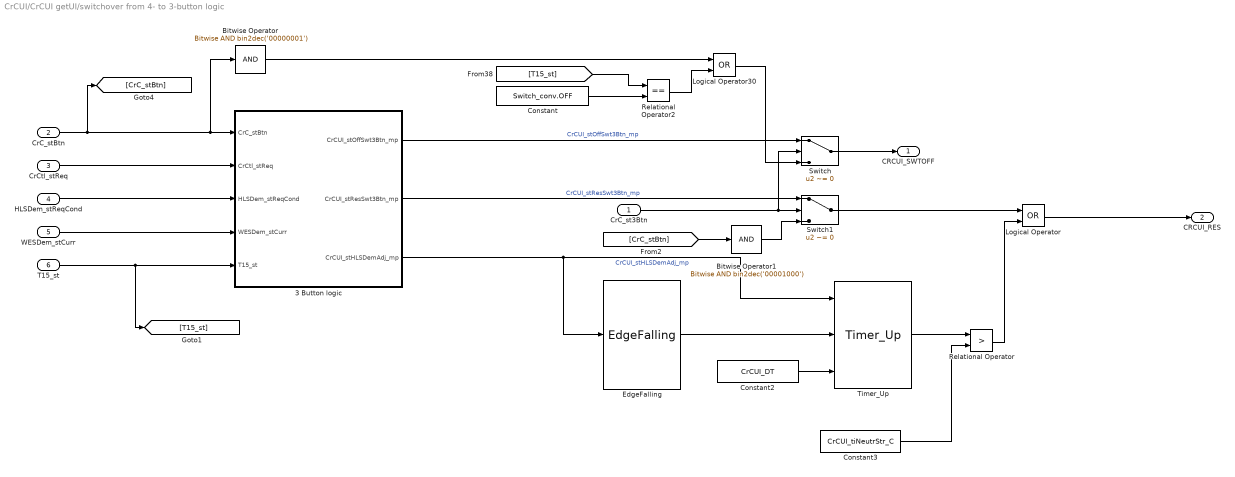
== system CrCUI/CrCUI getUI/switchover from 4- to 3-button logic ==
  CrC_st3Btn : Inport
  CrC_stBtn : Inport  Port=2
  CrCtl_stReq : Inport  Port=3
  HLSDem_stReqCond : Inport  Port=4
  WESDem_stCurr : Inport  Port=5
  T15_st : Inport  Port=6
  3 Button logic : Subsystem
  Bitwise Operator : simulink/Logic and Bit Operations/Bitwise Operator  logicop=AND  UseBitMask=on  BitMask=bin2dec('00000001')  BitMaskRealWorld=Stored Integer
  Bitwise Operator1 : simulink/Logic and Bit Operations/Bitwise Operator  logicop=AND  UseBitMask=on  BitMask=bin2dec('00001000')  BitMaskRealWorld=Stored Integer
  Constant : Constant  Value=Switch_conv.OFF
  Constant2 : Constant  Value=CrCUI_DT
  Constant3 : Constant  Value=CrCUI_tiNeutrStr_C
  EdgeFalling : CXLib/EdgeFalling
  Logical Operator : Logic  Operator=OR  AllPortsSameDT=off  OutDataTypeStr=boolean
  Logical Operator30 : Logic  Operator=OR  AllPortsSameDT=off  OutDataTypeStr=boolean
  Relational Operator : RelationalOperator  Operator=>  OutDataTypeStr=boolean  RndMeth=Simplest
  Relational Operator2 : RelationalOperator  Operator===  OutDataTypeStr=boolean  RndMeth=Simplest
  Switch : Switch  Criteria=u2 ~= 0
  Switch1 : Switch  Criteria=u2 ~= 0
  Timer_Up : CXLib/Timer_Up
  CRCUI_SWTOFF : Outport
  CRCUI_RES : Outport  Port=2
  wires:
  [T15_st] -> Relational Operator2/1
  CrC_stBtn/1 -> [CrC_stBtn], Bitwise Operator/1, 3 Button logic/1(CrC_stBtn)
  Bitwise Operator/1 -> Logical Operator30/1
  WESDem_stCurr/1 -> 3 Button logic/4(WESDem_stCurr)
  EdgeFalling/1 -> Timer_Up/2
  Constant2/1 -> Timer_Up/3
  Switch1/1 -> Logical Operator/1
  Constant3/1 -> Relational Operator/2
  3 Button logic/1(CrCUI_stOffSwt3Btn_mp) -> Switch/1  "CrCUI_stOffSwt3Btn_mp"
  Switch/1 -> CRCUI_SWTOFF/1
  CrC_st3Btn/1 -> Switch/2, Switch1/2
  Relational Operator/1 -> Logical Operator/2
  CrCtl_stReq/1 -> 3 Button logic/2(CrCtl_stReq)
  HLSDem_stReqCond/1 -> 3 Button logic/3(HLSDem_stReqCond)
  Bitwise Operator1/1 -> Switch1/3
  Timer_Up/1 -> Relational Operator/1
  Relational Operator2/1 -> Logical Operator30/2
  Logical Operator30/1 -> Switch/3
  T15_st/1 -> [T15_st], 3 Button logic/5(T15_st)
  Logical Operator/1 -> CRCUI_RES/1
  [CrC_stBtn] -> Bitwise Operator1/1
  3 Button logic/2(CrCUI_stResSwt3Btn_mp) -> Switch1/1  "CrCUI_stResSwt3Btn_mp"
  3 Button logic/3(CrCUI_stHLSDemAdj_mp) -> EdgeFalling/1, Timer_Up/1  "CrCUI_stHLSDemAdj_mp"
  Constant/1 -> Relational Operator2/2

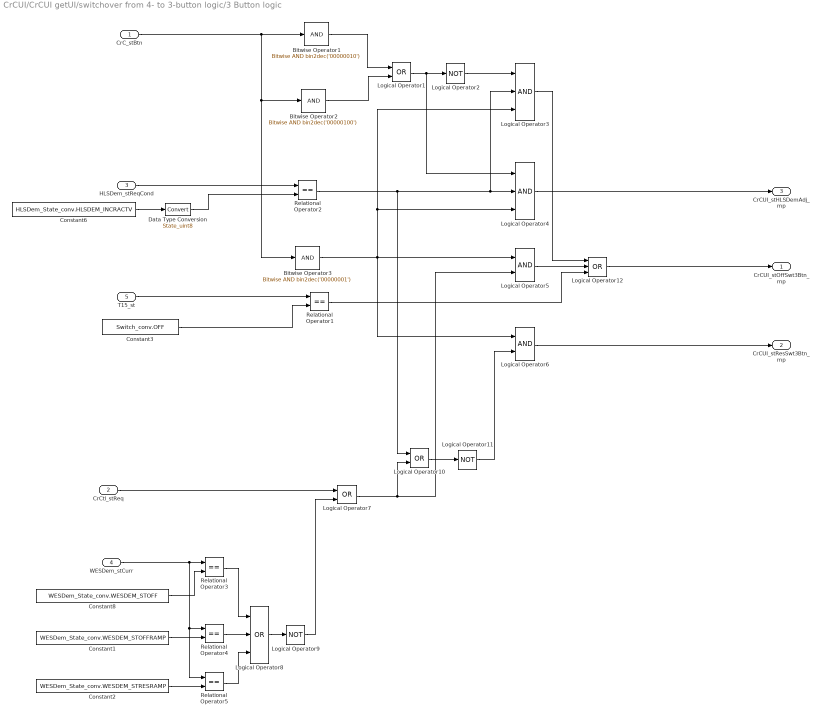
== system CrCUI/CrCUI getUI/switchover from 4- to 3-button logic/3 Button logic ==
  CrC_stBtn : Inport
  CrCtl_stReq : Inport  Port=2
  HLSDem_stReqCond : Inport  Port=3
  WESDem_stCurr : Inport  Port=4
  T15_st : Inport  Port=5
  Bitwise Operator1 : simulink/Logic and Bit Operations/Bitwise Operator  logicop=AND  UseBitMask=on  BitMask=bin2dec('00000010')  BitMaskRealWorld=Stored Integer
  Bitwise Operator2 : simulink/Logic and Bit Operations/Bitwise Operator  logicop=AND  UseBitMask=on  BitMask=bin2dec('00000100')  BitMaskRealWorld=Stored Integer
  Bitwise Operator3 : simulink/Logic and Bit Operations/Bitwise Operator  logicop=AND  UseBitMask=on  BitMask=bin2dec('00000001')  BitMaskRealWorld=Stored Integer
  Constant1 : Constant  Value=WESDem_State_conv.WESDEM_STOFFRAMP
  Constant2 : Constant  Value=WESDem_State_conv.WESDEM_STRESRAMP
  Constant3 : Constant  Value=Switch_conv.OFF
  Constant6 : Constant  Value=HLSDem_State_conv.HLSDEM_INCRACTV
  Constant8 : Constant  Value=WESDem_State_conv.WESDEM_STOFF
  Data Type Conversion : DataTypeConversion  OutDataTypeStr=State_uint8
  Logical Operator1 : Logic  Operator=OR  AllPortsSameDT=off  OutDataTypeStr=boolean
  Logical Operator10 : Logic  Operator=OR  AllPortsSameDT=off  OutDataTypeStr=boolean
  Logical Operator11 : Logic  Operator=NOT  AllPortsSameDT=off  OutDataTypeStr=boolean
  Logical Operator12 : Logic  Operator=OR  Inputs=3  AllPortsSameDT=off  OutDataTypeStr=boolean
  Logical Operator2 : Logic  Operator=NOT  AllPortsSameDT=off  OutDataTypeStr=boolean
  Logical Operator3 : Logic  Inputs=3  AllPortsSameDT=off  OutDataTypeStr=boolean
  Logical Operator4 : Logic  Inputs=3  AllPortsSameDT=off  OutDataTypeStr=boolean
  Logical Operator5 : Logic  AllPortsSameDT=off  OutDataTypeStr=boolean
  Logical Operator6 : Logic  AllPortsSameDT=off  OutDataTypeStr=boolean
  Logical Operator7 : Logic  Operator=OR  AllPortsSameDT=off  OutDataTypeStr=boolean
  Logical Operator8 : Logic  Operator=OR  Inputs=3  AllPortsSameDT=off  OutDataTypeStr=boolean
  Logical Operator9 : Logic  Operator=NOT  AllPortsSameDT=off  OutDataTypeStr=boolean
  Relational Operator{1..5} (5 alike) : RelationalOperator  Operator===  OutDataTypeStr=boolean  RndMeth=Simplest
  CrCUI_stOffSwt3Btn_mp : Outport
  CrCUI_stResSwt3Btn_mp : Outport  Port=2
  CrCUI_stHLSDemAdj_mp : Outport  Port=3
  wires:
  Bitwise Operator1/1 -> Logical Operator1/1
  Bitwise Operator2/1 -> Logical Operator1/2
  Logical Operator1/1 -> Logical Operator4/1, Logical Operator2/1
  Logical Operator2/1 -> Logical Operator3/1
  HLSDem_stReqCond/1 -> Relational Operator2/1
  Constant6/1 -> Data Type Conversion/1
  Relational Operator2/1 -> Logical Operator4/2, Logical Operator3/2, Logical Operator10/1
  CrC_stBtn/1 -> Bitwise Operator3/1, Bitwise Operator2/1, Bitwise Operator1/1
  Bitwise Operator3/1 -> Logical Operator6/1, Logical Operator5/1, Logical Operator4/3, Logical Operator3/3
  CrCtl_stReq/1 -> Logical Operator7/1
  WESDem_stCurr/1 -> Relational Operator5/1, Relational Operator4/1, Relational Operator3/1
  Constant8/1 -> Relational Operator3/2
  Constant1/1 -> Relational Operator4/2
  Relational Operator4/1 -> Logical Operator8/2
  Relational Operator3/1 -> Logical Operator8/1
  Relational Operator5/1 -> Logical Operator8/3
  Logical Operator8/1 -> Logical Operator9/1
  Logical Operator9/1 -> Logical Operator7/2
  Logical Operator7/1 -> Logical Operator5/2, Logical Operator10/2
  Logical Operator10/1 -> Logical Operator11/1
  Logical Operator11/1 -> Logical Operator6/2
  Logical Operator5/1 -> Logical Operator12/2
  Logical Operator3/1 -> Logical Operator12/1
  Logical Operator4/1 -> CrCUI_stHLSDemAdj_mp/1
  Logical Operator6/1 -> CrCUI_stResSwt3Btn_mp/1
  Logical Operator12/1 -> CrCUI_stOffSwt3Btn_mp/1
  T15_st/1 -> Relational Operator1/1
  Relational Operator1/1 -> Logical Operator12/3
  Constant2/1 -> Relational Operator5/2
  Constant3/1 -> Relational Operator1/2
  Data Type Conversion/1 -> Relational Operator2/2
